simulink model "Iris_DeePC_Control_Gazebo_MPC_aux_linear"  (R2022a)
settings: Solver=VariableStepAuto  StartTime=0.0  StopTime=sim_time  RelTol=1e-3
values from neighbouring files (symbols this model uses):
  Ad = param.Ad_sys    [DeePC_main.m]    (also in MPC_main.m = param.Ad_MPC; ex_MPC_code.m = param.Ad_MPC)
  Bd = param.Bd_sys    [DeePC_main.m]    (also in MPC_main.m = param.Bd_MPC; ex_MPC_code.m = param.Bd_MPC)
  K_mpc = Rt^(-1)*St*Fb    [MPC_main.m]
  K_pitch = param.K_lqr_outer_loop(3,8)    [DeePC_main.m]    (also in MPC_main.m)
  K_roll = param.K_lqr_outer_loop(2,7)    [DeePC_main.m]    (also in MPC_main.m)
  K_yaw = param.K_lqr_outer_loop(4,9)    [DeePC_main.m]    (also in MPC_main.m)
  Ky_mpc = Rt^(-1)*St    [MPC_main.m]
  N_mpc = Nd    (= 50)    [MPC_main.m]
  nu_mpc = size(Bd_mpc,2)    [MPC_main.m]
  param = load_crazyflie_parameters()    [DeePC_main.m]    (also in MPC_Optimizer.m = evalin('base', 'param'); MPC_main.m; ex_MPC_code.m)
  start_time = 2    [DeePC_main.m]    (also in MPC_main.m = 0)
  wave_time = 10    [MPC_main.m]
undefined symbols (not defined in the file or in its folder): MPC_Optimizer, Yb_mpc
libraries: Crazyflie_Library x1
settings Model: Creator=ezzat  LastModifiedBy=simao
settings SolverCC: AlgebraicLoopSolver=LineSearch
settings DataIOCC: ReturnWorkspaceOutputs=off
settings DebuggingCC: UnconnectedInputMsg=warning  UnconnectedOutputMsg=warning  UnconnectedLineMsg=warning  SFMachineParentedDataDiag=warning  ArithmeticOperatorsInVariantConditions=warning
settings SFSimCC: CustomCodeUndefinedFunction=UseInterfaceOnly

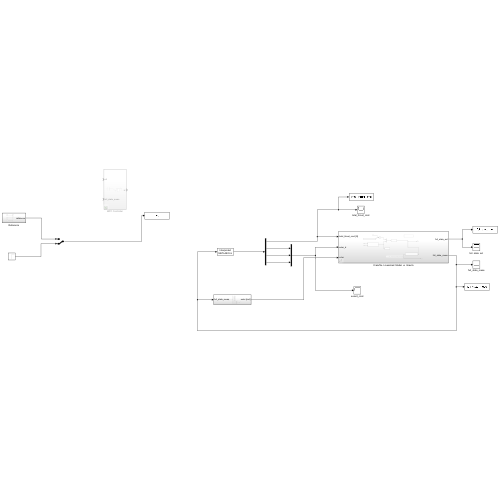
[thumbnail: Simulink's stored preview of the top-level diagram]
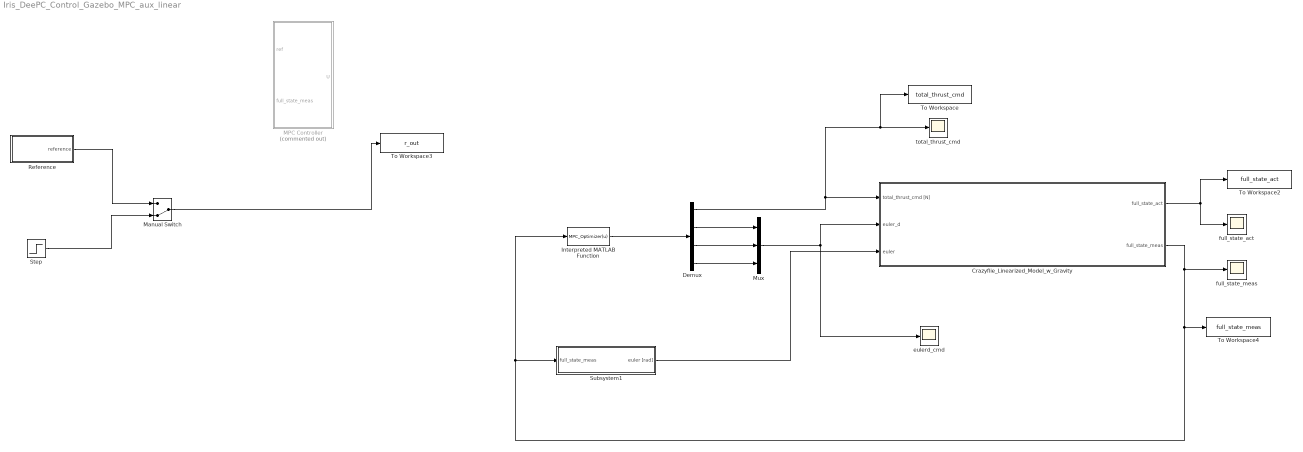
== system Iris_DeePC_Control_Gazebo_MPC_aux_linear ==
  Crazyflie_Linearized_Model_w_Gravity : Subsystem  AncestorBlock=Crazyflie_Library/Crazyflie_Linearized_Model_w_Gravity
  Demux : Demux
  Interpreted MATLAB Function : MATLABFcn  MATLABFcn=MPC_Optimizer(u)  OutputDimensions=4
  MPC Controller : Subsystem  Commented=on
  Manual Switch : ManualSwitch  CurrentSetting=0
  Mux : Mux  Inputs=3
  Reference : Subsystem
  Step : Step  Time=start_time  Before=[param.nrotor_initial_condition(1:3); param.nrotor_initial_condition(9)]  After=[param.nrotor_final_condition(1:3); param.nrotor_final_condition(9)]  SampleTime=0
  Subsystem1 : Subsystem
  To Workspace : ToWorkspace  VariableName=total_thrust_cmd  SampleTime=param.sample_time_controller_outer
  To Workspace2 : ToWorkspace  VariableName=full_state_act  SampleTime=param.sample_time_controller_outer
  To Workspace3 : ToWorkspace  VariableName=r_out  SampleTime=param.sample_time_controller_outer
  To Workspace4 : ToWorkspace  VariableName=full_state_meas  SampleTime=param.sample_time_controller_outer
  eulerd_cmd : Scope
  full_state_act : Scope
  full_state_meas : Scope
  total_thrust_cmd : Scope
  wires:
  Crazyflie_Linearized_Model_w_Gravity/1(full_state_act) -> full_state_act/1, To Workspace2/1
  Step/1 -> Manual Switch/2
  Reference/1(reference) -> Manual Switch/1
  Manual Switch/1 -> To Workspace3/1
  Demux/2 -> Mux/1
  Demux/3 -> Mux/2
  Demux/4 -> Mux/3
  Demux/1 -> To Workspace/1, total_thrust_cmd/1, Crazyflie_Linearized_Model_w_Gravity/1(total_thrust_cmd [N])
  Mux/1 -> Crazyflie_Linearized_Model_w_Gravity/2(euler_d), eulerd_cmd/1
  Interpreted MATLAB Function/1 -> Demux/1
  Crazyflie_Linearized_Model_w_Gravity/2(full_state_meas) -> To Workspace4/1, Subsystem1/1(full_state_meas), Interpreted MATLAB Function/1, full_state_meas/1
  Subsystem1/1(euler [rad]) -> Crazyflie_Linearized_Model_w_Gravity/3(euler)

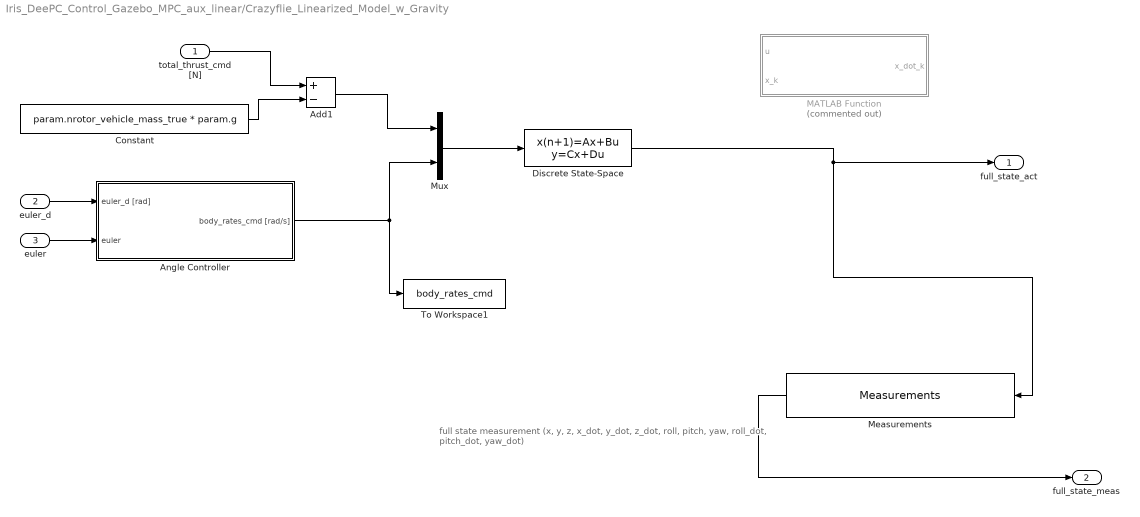
== system Iris_DeePC_Control_Gazebo_MPC_aux_linear/Crazyflie_Linearized_Model_w_Gravity ==
  note: full state measurement
      | (x, y, z, x_dot, y_dot, z_dot, roll, pitch, yaw, roll_dot, pitch_dot, yaw_dot)
  total_thrust_cmd [N] : Inport
  euler_d : Inport  Port=2
  euler : Inport  Port=3
  Add1 : Sum  Inputs=+-
  Angle Controller : Subsystem
  Constant : Constant  Value=param.nrotor_vehicle_mass_true * param.g
  Discrete State-Space : DiscreteStateSpace  A=param.Ad_MPC  B=param.Bd_MPC  C=param.Cd_MPC  D=zeros(9,4)  InitialCondition=param.nrotor_initial_condition(1:9)  SampleTime=0.04
  MATLAB Function : MATLAB Function  Commented=on  TreatAsAtomicUnit=on
  Measurements : Crazyflie_Library/Crazyflie_Linearized_Model_w_Gravity/Measurements  SystemSampleTime=-1  VariantActivationTime=update diagram  Latency=0  AutoFrameSizeCalculation=off
  Mux : Mux  Inputs=2
  To Workspace1 : ToWorkspace  VariableName=body_rates_cmd  SampleTime=param.sample_time_controller_outer
  full_state_act : Outport  VectorParamsAs1DForOutWhenUnconnected=off
  full_state_meas : Outport  Port=2  VectorParamsAs1DForOutWhenUnconnected=off
  wires:
  Discrete State-Space/1 -> Measurements/1, full_state_act/1
  total_thrust_cmd [N]/1 -> Add1/1
  Add1/1 -> Mux/1
  Constant/1 -> Add1/2
  Measurements/1 -> full_state_meas/1
  Angle Controller/1(body_rates_cmd [rad/s]) -> Mux/2, To Workspace1/1
  Mux/1 -> Discrete State-Space/1
  euler_d/1 -> Angle Controller/1(euler_d [rad])
  euler/1 -> Angle Controller/2(euler)

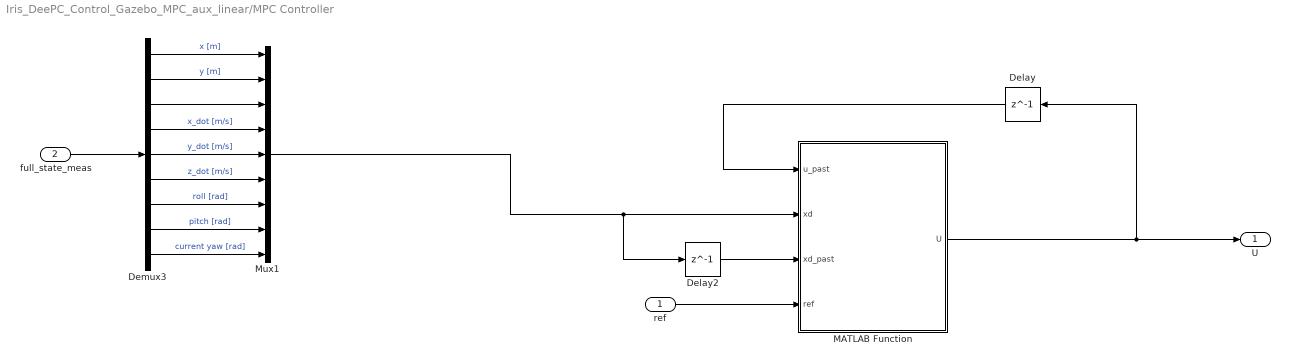
== system Iris_DeePC_Control_Gazebo_MPC_aux_linear/MPC Controller ==
  ref : Inport
  full_state_meas : Inport  Port=2
  Delay : Delay  DelayLength=1  InitialCondition=zeros(4,1)
  Delay2 : Delay  DelayLength=1  InitialCondition=zeros(9,1)
  Demux3 : Demux  Outputs=9
  MATLAB Function : MATLAB Function  TreatAsAtomicUnit=on
  Mux1 : Mux  Inputs=9
  U : Outport
  wires:
  MATLAB Function/1(U) -> Delay/1, U/1
  ref/1 -> MATLAB Function/4(ref)
  Delay/1 -> MATLAB Function/1(u_past)
  Delay2/1 -> MATLAB Function/3(xd_past)
  full_state_meas/1 -> Demux3/1
  Demux3/1 -> Mux1/1  "x [m]"
  Demux3/2 -> Mux1/2  "y [m]"
  Demux3/3 -> Mux1/3
  Demux3/4 -> Mux1/4  "x_dot [m/s]"
  Demux3/5 -> Mux1/5  "y_dot [m/s]"
  Demux3/6 -> Mux1/6  "z_dot [m/s]"
  Demux3/7 -> Mux1/7  "roll [rad]"
  Demux3/8 -> Mux1/8  "pitch [rad]"
  Demux3/9 -> Mux1/9  "current yaw [rad]"
  Mux1/1 -> Delay2/1, MATLAB Function/2(xd)

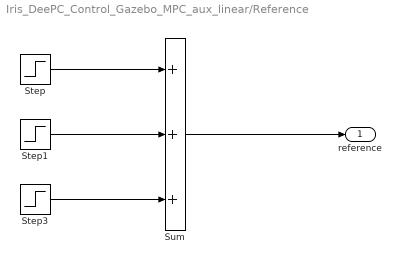
== system Iris_DeePC_Control_Gazebo_MPC_aux_linear/Reference ==
  Step : Step  Time=start_time  Before=[param.nrotor_initial_condition(1:3); param.nrotor_initial_condition(9)]  After=[param.nrotor_final_condition(1:3); param.nrotor_final_condition(9)]  SampleTime=0
  Step1 : Step  Time=start_time+wave_time  Before=[0;0;0;0]  After=[-1;-1;1;0]  SampleTime=0
  Step3 : Step  Time=start_time+wave_time*2  Before=[0;0;0;0]  After=[1;1;-1;0]  SampleTime=0
  Sum : Sum  Inputs=+++
  reference : Outport
  wires:
  Sum/1 -> reference/1
  Step/1 -> Sum/1
  Step1/1 -> Sum/2
  Step3/1 -> Sum/3

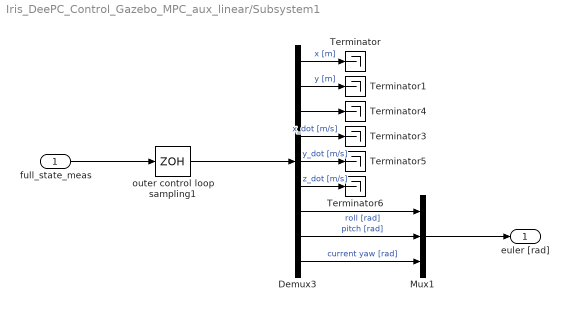
== system Iris_DeePC_Control_Gazebo_MPC_aux_linear/Subsystem1 ==
  full_state_meas : Inport
  Demux3 : Demux  Outputs=9
  Mux1 : Mux  Inputs=3
  Terminator{,1,3..6} (6 alike) : Terminator
  outer control loop sampling1 : ZeroOrderHold  SampleTime=param.sample_time_controller_outer
  euler [rad] : Outport
  wires:
  Demux3/7 -> Mux1/1  "roll [rad]"
  outer control loop sampling1/1 -> Demux3/1
  Demux3/8 -> Mux1/2  "pitch [rad]"
  full_state_meas/1 -> outer control loop sampling1/1
  Demux3/9 -> Mux1/3  "current yaw [rad]"
  Mux1/1 -> euler [rad]/1
  Demux3/1 -> Terminator/1  "x [m]"
  Demux3/2 -> Terminator1/1  "y [m]"
  Demux3/3 -> Terminator4/1
  Demux3/4 -> Terminator3/1  "x_dot [m/s]"
  Demux3/5 -> Terminator5/1  "y_dot [m/s]"
  Demux3/6 -> Terminator6/1  "z_dot [m/s]"

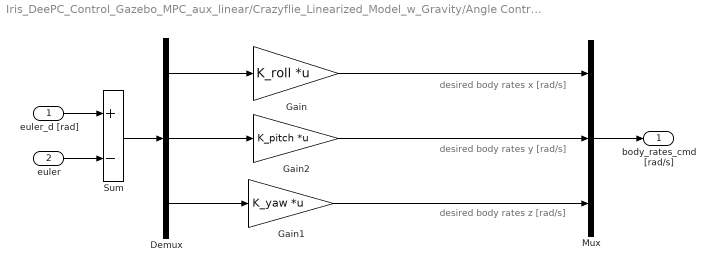
== system Iris_DeePC_Control_Gazebo_MPC_aux_linear/Crazyflie_Linearized_Model_w_Gravity/Angle Controller ==
  note: desired body rates x [rad/s]
  note: desired body rates z [rad/s]
  note: desired body rates y [rad/s]
  euler_d [rad] : Inport
  euler : Inport  Port=2
  Demux : Demux  Outputs=3
  Gain : Gain  Gain=K_roll  Multiplication=Matrix(K*u)
  Gain1 : Gain  Gain=K_yaw  Multiplication=Matrix(K*u)
  Gain2 : Gain  Gain=K_pitch  Multiplication=Matrix(K*u)
  Mux : Mux  Inputs=3
  Sum : Sum  Inputs=+-
  body_rates_cmd [rad/s] : Outport
  wires:
  euler_d [rad]/1 -> Sum/1
  euler/1 -> Sum/2
  Demux/2 -> Gain2/1
  Demux/3 -> Gain1/1
  Mux/1 -> body_rates_cmd [rad/s]/1
  Sum/1 -> Demux/1
  Gain2/1 -> Mux/2
  Gain1/1 -> Mux/3
  Gain/1 -> Mux/1
  Demux/1 -> Gain/1

== matlab function Iris_DeePC_Control_Gazebo_MPC_aux_linear/Crazyflie_Linearized_Model_w_Gravity/MATLAB Function ==
  settings: updateMethod=DISCRETE  sampleTime=0.04
  data: u input; x_dot_k output; x_k input; Ad parameter; Bd parameter
function x_dot_k = fcn(u,x_k, Ad, Bd)

x_dot_k = zeros(9,1);

x_dot_k = Ad*x_k + Bd*u;

== matlab function Iris_DeePC_Control_Gazebo_MPC_aux_linear/MPC Controller/MATLAB Function ==
  settings: updateMethod=DISCRETE  sampleTime=0.04
  data: u_past input; U output; xd input; xd_past input; ref input; Ky_mpc parameter; N_mpc parameter; K_mpc parameter; nu_mpc parameter; Yb_mpc parameter
function U  = MPC_otimizer(u_past,xd,xd_past,ref,Ky_mpc,N_mpc, K_mpc, nu_mpc,Yb_mpc)

U = zeros(4,1);
% Yb_mpc2 = zeros(0,0);
Cd = eye(9);

% for n = 0:N_mpc
%     Yb_mpc2 =[Yb_mpc2;ref];
% end


Dxdk = xd-xd_past;
xk = [ Dxdk; Cd*xd];

% compute unconstrained optimal sequence and MPC policy
dU = reshape(- (K_mpc*xk - Ky_mpc*Yb_mpc) , nu_mpc, N_mpc);
Uopt = u_past + dU;
U = Uopt(:,1);
